simulink model "R7014E_Measure"  (R2018a)
settings: Solver=ode5  StartTime=0.0  StopTime=inf  RelTol=1e-3  EnableMultiTasking=on
values from neighbouring files (symbols this model uses):
  A = [a_1*(-1/sqrt(2*g*(h1+EqPoint))) 0 ... (first row only)    [myTank.m]
  B = [6.95/36.2; 0]    [myTank.m]
  C = [0 1]    [myTank.m]
  EqPoint = 7    [myTank.m]
  K = (P*C' + N*0)/[0 1]    [myTank.m]
undefined symbols (not defined in the file or in its folder): National_Instruments, PCI
libraries: sldrtlib x2
settings Model: Creator=wolfgang  LastModifiedBy=anttib-5
settings Model: ModifiedHistory=|
  | Created an adjusted empty Simulink diagram for the lab assignments
  | in the course R0002E
settings SolverCC: AutoInsertRateTranBlk=on
settings DataIOCC: SaveFormat=Array  SignalLoggingSaveFormat=ModelDataLogs  SaveOutput=off  SignalLogging=off  DSMLogging=off  SaveTime=off
settings OptimizationCC: ExpressionDepthLimit=2147483647  LifeSpan=inf
settings DebuggingCC: UnderspecifiedInitializationDetection=Classic  MergeDetectMultiDrivingBlocksExec=none  SolverPrmCheckMsg=warning  FcnCallInpInsideContextMsg=warning  StateNameClashWarn=warning  SFUnexpectedBacktrackingDiag=warning  SFNoUnconditionalDefaultTransitionDiag=warning  SFExecutionAtInitializationDiag=none
settings HardwareCC: ProdBitPerPointer=32  ProdBitPerSizeT=32  ProdBitPerPtrDiffT=32  ProdLargestAtomicFloat=None  ProdIntDivRoundTo=Undefined  ProdEndianess=Unspecified  ProdWordSize=32  ProdHWDeviceType=32-bit Generic
settings ModelReferenceCC: PropagateSignalLabelsOutOfModel=off
settings CodeAppCC: StateflowObjectComments=on
settings GRTTargetCC: TargetLangStandard=C89/C90 (ANSI)  GeneratePreprocessorConditionals=Disable all
settings ConfigComp: CovMetricSettings=dw  CovHtmlReporting=on  CovSaveCumulativeToWorkspaceVar=on  CovSaveSingleToWorkspaceVar=on  CovExternalEMLEnable=off  CovSFcnEnable=off

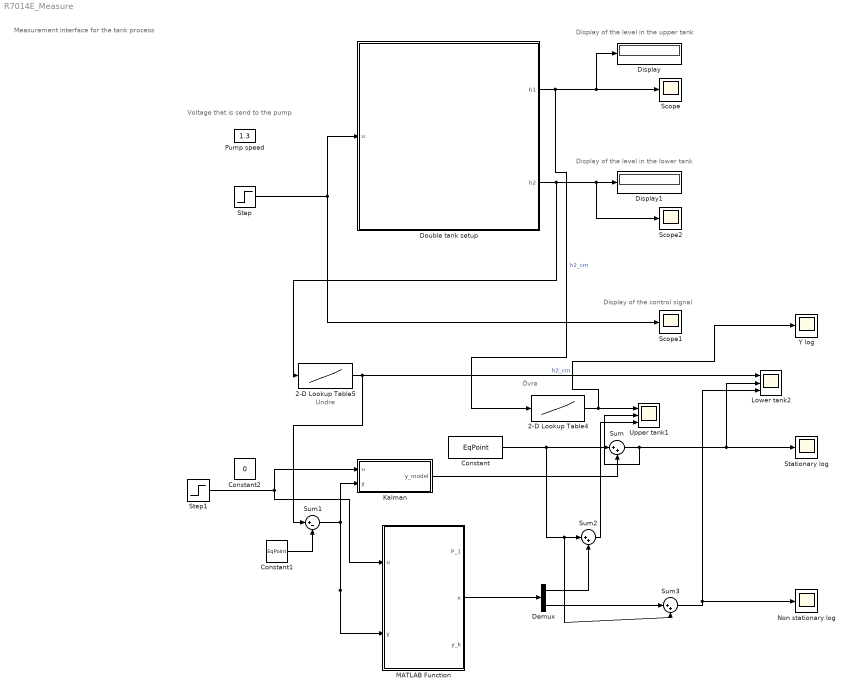
== system R7014E_Measure ==
  note: Undre
  note: Övre
  note: Measurement interface for the tank process
  note: Voltage that is send to the pump
  note: Display of the level in the upper tank
  note: Display of the control signal
  note: Display of the level in the lower tank
  2-D Lookup Table4 : Lookup_n-D  NumberOfTableDimensions=1  BreakpointsForDimension1=x  BreakpointsForDimension2=[1:3]  Table=y  RndMeth=Simplest  InputSameDT=on  mask{x=[0, 0.90, 2.17, 3.54, 4.79, 5.9, 6.997, 7.78, 8.53, 9.395, 9.995], y=[0, 3.4, 5, 6.8, 8.4, 9.7, 11, 12, 13, 14.2, 15.1]}
      mask prompts: x "Values on x-axis"; y "Values on y-axis"
  2-D Lookup Table5 : Lookup_n-D  NumberOfTableDimensions=1  BreakpointsForDimension1=x  BreakpointsForDimension2=[1:3]  Table=y  RndMeth=Simplest  InputSameDT=on  mask{x=[0, 0.811, 2.856, 3.374, 4.058, 4.839, 5.615, 6.475, 7.432, 8.174, 8.838], y=[0, 6.1, 6.8, 7.5, 8.6, 9.5, 10.7, 11.7, 13.1, 13.7, 14.9]}
      mask prompts: x "Values on x-axis"; y "Values on y-axis"
  Constant : Constant  Value=EqPoint
  Constant1 : Constant  Value=EqPoint
  Constant2 : Constant  Value=0
  Demux : Demux  Outputs=2
  Display : Display
  Display1 : Display
  Double tank setup : Subsystem  AncestorBlock=R0002E_lib/Double tank setup  StopFcn=|  mask(Realtime interface for the tank process){ts=0.02, h1_ch=0, h2_ch=1, u_ch=0}
      | chn =get_param(gcb,'u_ch');                          
      | s = daq.createSession('ni');                         
      | channel = ['ao',chn];                                
      | s.addAnalogOutputChannel('Dev1', channel, 'Voltage');
      | x = zeros(5,1);                                      
      | s.queueOutputData(x);                                
      | lh = s.addlistener('DataRequired', ...               
      | @(src,event) src.queueOutputData(x));                
      | s.startBackground();                                 
      | s.wait();                                            
      | s.stop();                                            
      | delete(lh);                                          
      | clear chn;                                           
      | clear s;                                             
      | clear channel;                                       
      | clear lh;                                            
      | clear x;
      mask prompts: ts "Sample time"; h1_ch "A/D Channel for upper tank"; h2_ch "A/D Channel for lower tank"; u_ch "D/A Channel for pump"
      mask help:
      | This block represents the physical interface from the computer to the tank process.
      |
      | The input u is the voltage that is provided for the pump, the output h1 is the measured level in the upper tank in [V] and the output h2 is the
      | measured level in the lower tank in [V].
      |
      | You need to provide the sample rate at which the voltage to the pump is updated and the level measurements are sampled. The sample rate should not be less than 0.02 seconds.
      mask Display:
      | x=363;
      | y=381;
      | image(imread('tank_icon.jpg'));
      | text(250/x,309/y,'Sensor');
      | text(260/x,169/y,'Sensor');
      | text(335/x,289/y,'A');
      | text(351/x,283/y,'D');
      | text(335/x,100/y,'A');
      | text(351/x,95/y,'D');
      | text(22/x,187/y,'A');
      | text(5/x,195/y,'D');
      | text(225/x,278/y,'h_1','texmode','on');
      | text(225/x,146/y,'h_2','texmode','on');
      | text(300/x,270/y,sprintf('AI-%d',h1_ch));
      | text(300/x,80/y,sprintf('AI-%d',h2_ch));
      | text(40/x,173/y,sprintf('AO-%d',u_ch));
  Kalman : Subsystem
  Lower tank2 : Scope  NumInputPorts=3
  MATLAB Function : MATLAB Function  TreatAsAtomicUnit=on
  "Non stationary log " : Scope
  Pump speed : Constant  Value=1.3
  Scope : Scope
  Scope1 : Scope
  Scope2 : Scope
  "Stationary log " : Scope
  Step : Step  Time=90  Before=1.3  After=1.5  SampleTime=0.1
  Step1 : Step  Time=90  After=0.2  SampleTime=0.02
  Sum : Sum  Inputs=|++
  Sum1 : Sum  Inputs=|+-
  Sum2 : Sum  Inputs=|++
  Sum3 : Sum  Inputs=|++
  Upper tank1 : Scope  NumInputPorts=3
  "Y log " : Scope
  wires:
  Double tank setup/1(h1) -> 2-D Lookup Table4/1, Display/1, Scope/1  "h2_cm"
  Constant1/1 -> Sum1/2
  2-D Lookup Table5/1 -> Sum1/1, Lower tank2/1  "h2_cm"
  Sum1/1 -> MATLAB Function/2(y), Kalman/2(y)
  Constant/1 -> Sum3/2, Sum2/1, Sum/1
  Kalman/1("y_model ") -> Sum/2
  2-D Lookup Table4/1 -> "Y log "/1, Upper tank1/1
  MATLAB Function/2(x) -> Demux/1
  Sum2/1 -> Upper tank1/3
  Demux/1 -> Sum2/2
  Double tank setup/2(h2) -> 2-D Lookup Table5/1, Scope2/1, Display1/1
  Sum/1 -> Upper tank1/2, Lower tank2/2, "Stationary log "/1
  Demux/2 -> Sum3/1
  Sum3/1 -> "Non stationary log "/1, Lower tank2/3
  Step1/1 -> MATLAB Function/1(u), Kalman/1(u)
  Step/1 -> Scope1/1, Double tank setup/1(u)

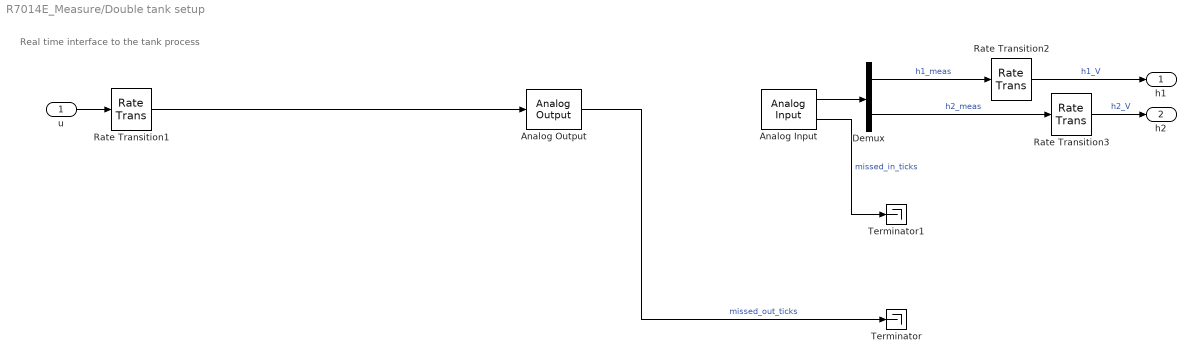
== system R7014E_Measure/Double tank setup ==
  note: Real time interface to the tank process
  u : Inport
  Analog Input : sldrtlib/Analog Input  SampleTime=ts  MaxMissedTicks=500000000  ShowMissedTicks=on  YieldWhenWaiting=off  DrvName=National_Instruments/PCI-6024E  DrvAddress=4294967295  DrvOptions=[0 0 0 0 0 0]  Channels=[h1_ch+1,h2_ch+1]  RangeMode=1  VoltRange=1  DataType=1
      settings: AttributesFormatString=National Instruments\nPCI-6024E [auto]  SourceProductName=Simulink Desktop Real-Time
  Analog Output : sldrtlib/Analog Output  SampleTime=ts  MaxMissedTicks=500000000  ShowMissedTicks=on  YieldWhenWaiting=off  DrvName=National_Instruments/PCI-6024E  DrvAddress=4294967295  DrvOptions=[0 0 0 0 0 0]  Channels=u_ch+1  RangeMode=1  VoltRange=1  InitialValue=0  FinalValue=0
      settings: AttributesFormatString=National Instruments\nPCI-6024E [auto]  SourceProductName=Simulink Desktop Real-Time
  Demux : Demux  Outputs=2
  Rate Transition1 : RateTransition  OutPortSampleTime=ts
  Rate Transition2 : RateTransition
  Rate Transition3 : RateTransition
  Terminator : Terminator
  Terminator1 : Terminator
  h1 : Outport
  h2 : Outport  Port=2
  wires:
  Rate Transition1/1 -> Analog Output/1
  Rate Transition3/1 -> h2/1  "h2_V"
  Rate Transition2/1 -> h1/1  "h1_V"
  Analog Input/2 -> Terminator1/1  "missed_in_ticks"
  Demux/2 -> Rate Transition3/1  "h2_meas"
  Demux/1 -> Rate Transition2/1  "h1_meas"
  Analog Input/1 -> Demux/1
  Analog Output/1 -> Terminator/1  "missed_out_ticks"
  u/1 -> Rate Transition1/1

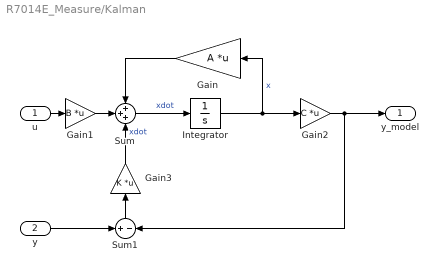
== system R7014E_Measure/Kalman ==
  u : Inport
  y : Inport  Port=2
  Gain : Gain  Gain=A  Multiplication=Matrix(K*u)
  Gain1 : Gain  Gain=B  Multiplication=Matrix(K*u)
  Gain2 : Gain  Gain=C  Multiplication=Matrix(K*u)
  Gain3 : Gain  Gain=K  Multiplication=Matrix(K*u)
  Integrator : Integrator
  Sum : Sum  Inputs=+++
  Sum1 : Sum  Inputs=+|-
  "y_model " : Outport
  wires:
  Sum/1 -> Integrator/1  "xdot"
  Integrator/1 -> Gain2/1, Gain/1  "x"
  Gain1/1 -> Sum/2
  u/1 -> Gain1/1
  Gain2/1 -> "y_model "/1, Sum1/2
  y/1 -> Sum1/1
  Sum1/1 -> Gain3/1
  Gain/1 -> Sum/1
  Gain3/1 -> Sum/3  "xdot"

== matlab function R7014E_Measure/MATLAB Function ==
  settings: updateMethod=DISCRETE
  data: u input; y input; P_1 output; x output; y_k output
function [P_1,x, y_k] = fcn(u,y)
persistent P_0;
 if isempty(P_0)
        P_0  = [73 73;73 73];
 end
 persistent A_k;
 if isempty(A_k)
        A_k  = [0.994625616518811 0;0.00535991554025889 0.994625616518811];
 end
  persistent B_k;
 if isempty(B_k)
        B_k  = [0.00191472575791366;5.15447758058602e-06];
 end
  persistent C_k;
 if isempty(C_k)
        C_k  = [0 1];
 end
 persistent N_k;
 if isempty(N_k)
        N_k  = [0 1];
 end
 persistent Q_k;
 if isempty(Q_k)
        Q_k  = [10 0;0 0.1];
 end
 persistent R_k;
 if isempty(R_k)
        R_k  = 1.5;
 end
persistent x_0;
 if isempty(x_0)
     x_0 = [0 ; 0];
 end
persistent k_0;
 if isempty(k_0)
    k_0 = 0;
 end
 
x_hat = A_k*x_0+B_k*u;
P = A_k*P_0*A_k'+N_k*Q_k*N_k';

K = P*C_k'*inv(C_k*P*C_k'+R_k);
y_k = y-C_k*x_hat;
x = x_hat+K*y_k;

P_1 = P-K*C_k*P;
P_0 = P_1;
